simulink model "sistema_electromagnetico"  (R2016b)
settings: Solver=VariableStepAuto  StartTime=0.0  StopTime=10.0  RelTol=1e-3
values from neighbouring files (symbols this model uses):
  Ld = 6.6    [c4ModeloCompleto.m]    (also in c4ModeloCompleto_var.m = 0.0066)
  Lq = 5.8    [c4ModeloCompleto.m]    (also in c4ModeloCompleto_var.m = 0.0058)
  Pp = 3    [c4ModeloCompleto.m]    (also in c4ModeloCompleto_var.m)
  Rs = 1.02    [c4ModeloCompleto_var.m]
undefined symbols (not defined in the file or in its folder): L0
settings Model: Creator=agustin  LastModifiedBy=agustin

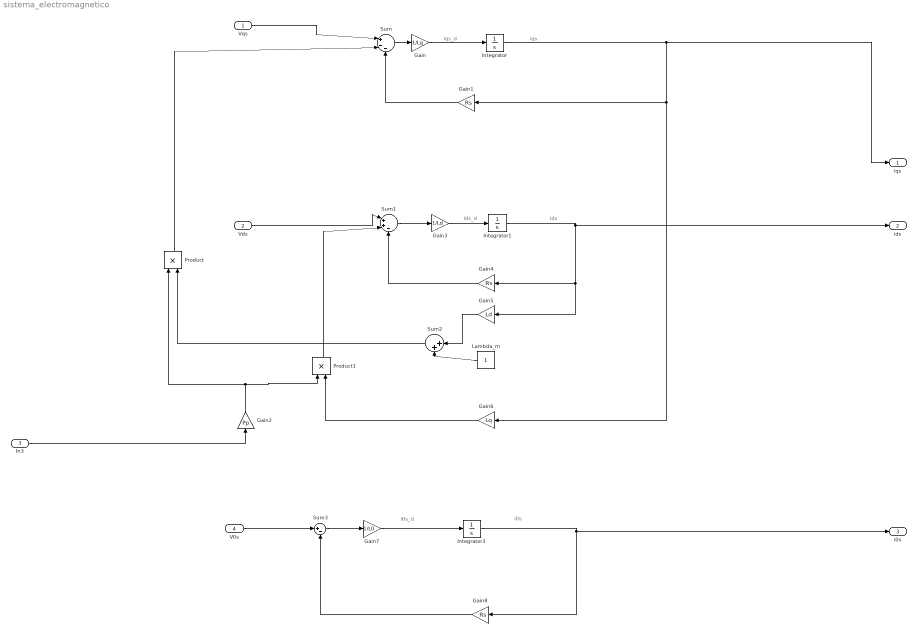
== system sistema_electromagnetico ==
  note: i0s
  note: i0s_d
  note: ids_d
  note: ids
  note: iqs
  note: iqs_d
  Vqs : Inport
  Vds : Inport  Port=2
  In3 : Inport  Port=3
  V0s : Inport  Port=4
  Gain : Gain  Gain=1/Lq
  Gain1 : Gain  Gain=Rs
  Gain2 : Gain  Gain=Pp
  Gain3 : Gain  Gain=1/Ld
  Gain4 : Gain  Gain=Rs
  Gain5 : Gain  Gain=Ld
  Gain6 : Gain  Gain=Lq
  Gain7 : Gain  Gain=1/L0
  Gain8 : Gain  Gain=Rs
  Integrator : Integrator
  Integrator1 : Integrator
  Integrator3 : Integrator
  "Lambda_m " : Constant
  Product : Product
  Product1 : Product
  Sum : Sum  Inputs=|+--
  Sum1 : Sum  Inputs=|++-
  Sum2 : Sum  Inputs=|++
  Sum3 : Sum  Inputs=|+-
  iqs : Outport
  ids : Outport  Port=2
  i0s : Outport  Port=3
  wires:
  Product/1 -> Sum/2
  In3/1 -> Gain2/1
  Product1/1 -> Sum1/2
  Gain2/1 -> Product1/1, Product/1
  V0s/1 -> Sum3/1
  Integrator/1 -> iqs/1, Gain1/1, Gain6/1
  Gain8/1 -> Sum3/2
  Sum2/1 -> Product/2
  Sum3/1 -> Gain7/1
  Vqs/1 -> Sum/1
  Sum/1 -> Gain/1
  Gain3/1 -> Integrator1/1
  Vds/1 -> Sum1/1
  Gain4/1 -> Sum1/3
  Integrator1/1 -> ids/1, Gain5/1, Gain4/1
  Sum1/1 -> Gain3/1
  Gain5/1 -> Sum2/1
  Gain/1 -> Integrator/1
  Gain6/1 -> Product1/2
  Gain1/1 -> Sum/3
  "Lambda_m "/1 -> Sum2/2
  Gain7/1 -> Integrator3/1
  Integrator3/1 -> i0s/1, Gain8/1
